simulink model "W09_1_vrx"  (R2024b)
settings: Solver=FixedStepDiscrete  StartTime=0.0  StopTime=inf  FixedStep=Ts_ctrl  RelTol=1e-3
values from neighbouring files (symbols this model uses):
  animate = 0    [W07_compare.m]    (also in W07_crab_demo.m; W07_lookahead_demo.m; W07_setup.m = 1; W09_setup.m = 1)
  crab_comp = 1    [W09_setup.m]
  Delta = DELTAS(i)    [W07_lookahead_demo.m]    (also in W07_setup.m = 10; W09_setup.m = 10)
  F_max = 500    [W07_setup.m]    (also in W09_setup.m)
  half_beam = 1.027135    [W07_setup.m]    (also in W09_setup.m)
  k_prop = 1000 * 0.004422 * 0.2^4    (= 0.0070752)    [W07_setup.m]    (also in W09_setup.m)
  Kd_psi = 200    [W07_setup.m]    (also in W09_setup.m)
  Ki_u = 100    [W07_setup.m]    (also in W09_setup.m)
  Kp_psi = 400    [W07_setup.m]    (also in W09_setup.m)
  Kp_u = 300    [W07_setup.m]    (also in W09_setup.m)
  loiter_radius = 18    [W09_setup.m]
  loiter_turns = 2    [W09_setup.m]
  loiter_wp = 3    [W09_setup.m]
  loiter_xc = wp_north(loiter_wp)    [W09_setup.m]
  loiter_yc = wp_east(loiter_wp)    [W09_setup.m]
  n_max = sqrt(F_max / k_prop)    [W07_setup.m]    (also in W09_setup.m)
  origin_east = -532    [W07_setup.m]    (also in W09_setup.m)
  origin_north = 162    [W07_setup.m]    (also in W09_setup.m)
  p_c = 0.313    [W09_setup.m]
  R_LOS = 5    [W07_lookahead_demo.m]    (also in W07_setup.m; W09_setup.m)
  tau_n = 0.30    (= 0.3)    [W07_setup.m]    (also in W09_setup.m)
  Ts_ctrl = 0.05    [W07_setup.m]    (also in W09_setup.m)
  u_ref = 1.5    [W07_setup.m]    (also in W09_setup.m)
  wp_east = [  20   20  100  100   20 ]    [W07_setup.m]    (also in W09_setup.m = [  20   20   55   90   90 ])
  wp_north = [ -20   60   60  -20  -20 ]    [W07_setup.m]    (also in W09_setup.m = [ -20   50   20   50  -20 ])
libraries: ros2lib x5, slpidlib x1
settings Model: Creator=admin  LastModifiedBy=admin

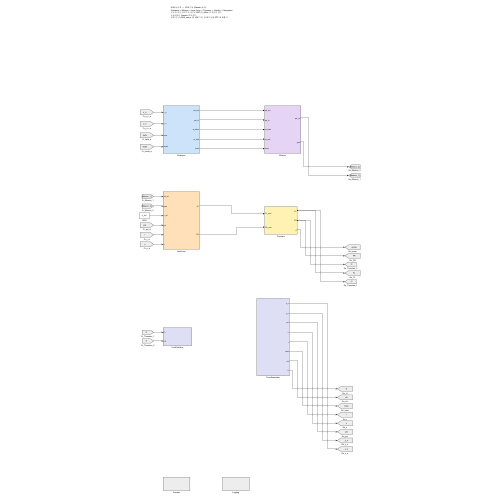
[thumbnail: Simulink's stored preview of the top-level diagram]
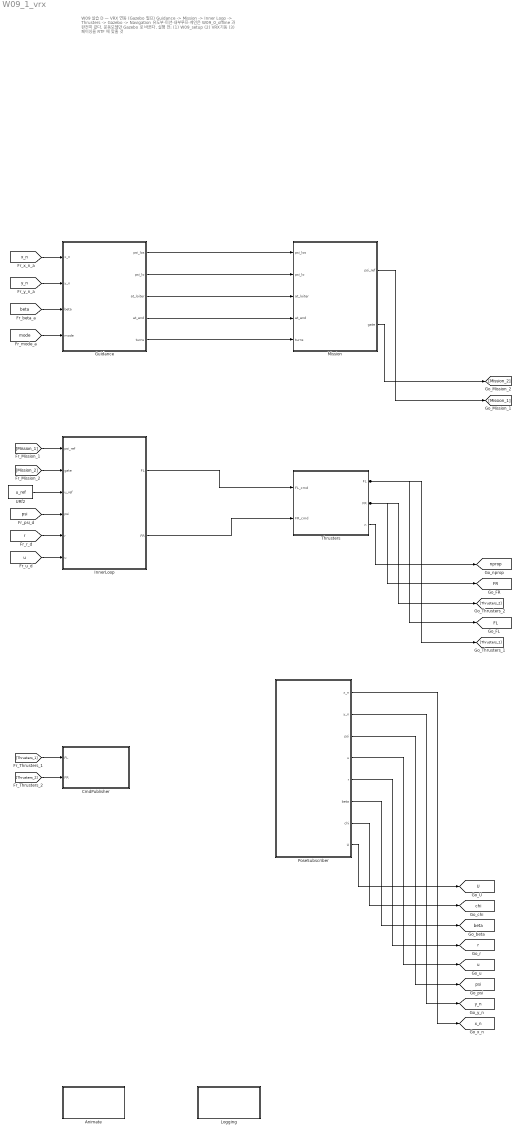
== system W09_1_vrx ==
  note: W09 실습 D  —  VRX 연동 (Gazebo 필요)
      | Guidance -> Mission -> Inner Loop -> Thrusters -> Gazebo -> Navigation
      | 유도부·미션·내부루프·게인은 W09_0_offline 과 완전히 같다.
      | 운동모델만 Gazebo 로 바뀐다.
      | 실행 전: (1) W09_setup  (2) VRX 기동  (3) 페이싱을 RTF 에 맞출 것
  Animate : Subsystem
  CmdPublisher : Subsystem
  Guidance : Subsystem
  InnerLoop : Subsystem
  Logging : Subsystem
  Mission : Subsystem
  PoseSubscriber : Subsystem
  Thrusters : Subsystem
  URf2 : Constant  Value=u_ref
  tag scope: FL=global, FR=global, U=global, beta=global, chi=global, nprop=global, psi=global, r=global, u=global, x_n=global, y_n=global
  wires:
  PoseSubscriber/8(U) -> [U]
  PoseSubscriber/7(chi) -> [chi]
  PoseSubscriber/6(beta) -> [beta]
  PoseSubscriber/5(r) -> [r]
  PoseSubscriber/4(u) -> [u]
  PoseSubscriber/3(psi) -> [psi]
  PoseSubscriber/2(y_n) -> [y_n]
  PoseSubscriber/1(x_n) -> [x_n]
  Thrusters/3(n) -> [nprop]
  Thrusters/2(FR) -> [FR], [Thrusters_2]
  Thrusters/1(FL) -> [FL], [Thrusters_1]
  InnerLoop/2(FR) -> Thrusters/2(FR_cmd)
  InnerLoop/1(FL) -> Thrusters/1(FL_cmd)
  [u] -> InnerLoop/6(u)
  [r] -> InnerLoop/5(r)
  [psi] -> InnerLoop/4(psi)
  URf2/1 -> InnerLoop/3(u_ref)
  Mission/2(gate) -> [Mission_2]
  Mission/1(psi_ref) -> [Mission_1]
  Guidance/5(turns) -> Mission/5(turns)
  Guidance/4(at_end) -> Mission/4(at_end)
  Guidance/3(at_loiter) -> Mission/3(at_loiter)
  Guidance/2(psi_lo) -> Mission/2(psi_lo)
  Guidance/1(psi_los) -> Mission/1(psi_los)
  [mode] -> Guidance/4(mode)
  [beta] -> Guidance/3(beta)
  [y_n] -> Guidance/2(y_n)
  [x_n] -> Guidance/1(x_n)
  [Thrusters_2] -> CmdPublisher/2(FR)
  [Thrusters_1] -> CmdPublisher/1(FL)
  [Mission_2] -> InnerLoop/2(gate)
  [Mission_1] -> InnerLoop/1(psi_ref)

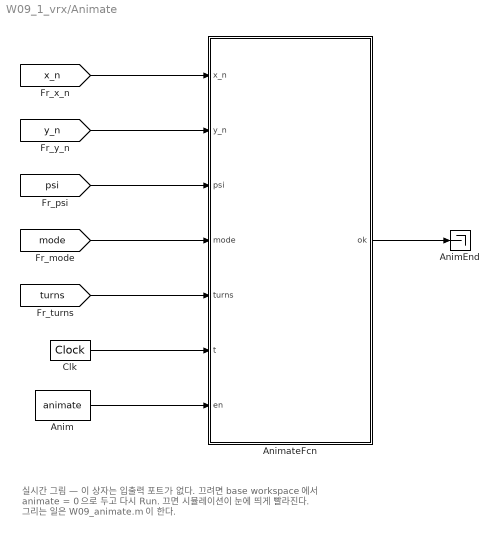
== system W09_1_vrx/Animate ==
  note: 실시간 그림 — 이 상자는 입출력 포트가 없다.
      | 끄려면 base workspace 에서  animate = 0  으로 두고 다시 Run.
      | 끄면 시뮬레이션이 눈에 띄게 빨라진다.
      | 그리는 일은 W09_animate.m 이 한다.
  Anim : Constant  Value=animate
  AnimEnd : Terminator
  AnimateFcn : MATLAB Function  TreatAsAtomicUnit=on
  Clk : DigitalClock  SampleTime=Ts_ctrl
  wires:
  [x_n] -> AnimateFcn/1(x_n)
  [y_n] -> AnimateFcn/2(y_n)
  [psi] -> AnimateFcn/3(psi)
  [mode] -> AnimateFcn/4(mode)
  [turns] -> AnimateFcn/5(turns)
  Clk/1 -> AnimateFcn/6(t)
  Anim/1 -> AnimateFcn/7(en)
  AnimateFcn/1(ok) -> AnimEnd/1

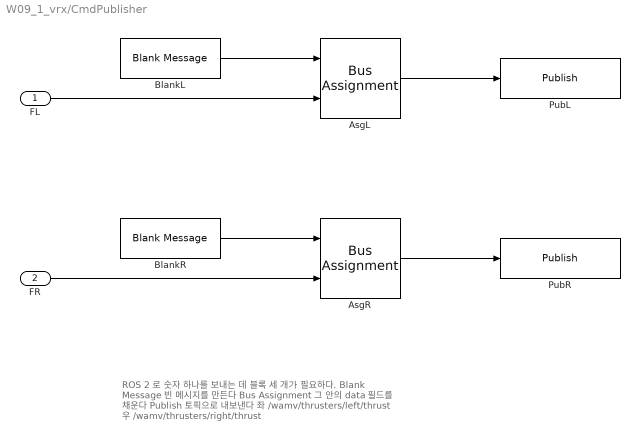
== system W09_1_vrx/CmdPublisher ==
  note: ROS 2 로 숫자 하나를 보내는 데 블록 세 개가 필요하다.
      |   Blank Message   빈 메시지를 만든다
      |   Bus Assignment  그 안의 data 필드를 채운다
      |   Publish         토픽으로 내보낸다
      |
      | 좌 /wamv/thrusters/left/thrust
      | 우 /wamv/thrusters/right/thrust
  FL : Inport
  FR : Inport  Port=2
  AsgL : BusAssignment  AssignedSignals=data
  AsgR : BusAssignment  AssignedSignals=data
  BlankL : ros2lib/Blank Message  messageClass=Message  entityType=std_msgs/Float64  messageType=std_msgs/Float64  SampleTime=Ts_ctrl
  BlankR : ros2lib/Blank Message  messageClass=Message  entityType=std_msgs/Float64  messageType=std_msgs/Float64  SampleTime=Ts_ctrl
  PubL : ros2lib/Publish  topicSource=Specify your own  topic=/wamv/thrusters/left/thrust  messageType=std_msgs/Float64  QOSHistory=Keep last  QOSDepth=1  QOSReliability=Reliable  QOSDurability=Volatile  QOSDeadline=Inf  QOSLifespan=Inf  QOSLiveliness=Automatic  QOSLeaseDuration=Inf  QOSAvoidROSNamespaceConventions=off
  PubR : ros2lib/Publish  topicSource=Specify your own  topic=/wamv/thrusters/right/thrust  messageType=std_msgs/Float64  QOSHistory=Keep last  QOSDepth=1  QOSReliability=Reliable  QOSDurability=Volatile  QOSDeadline=Inf  QOSLifespan=Inf  QOSLiveliness=Automatic  QOSLeaseDuration=Inf  QOSAvoidROSNamespaceConventions=off
  wires:
  BlankL/1 -> AsgL/1
  AsgL/1 -> PubL/1
  FL/1 -> AsgL/2
  BlankR/1 -> AsgR/1
  AsgR/1 -> PubR/1
  FR/1 -> AsgR/2

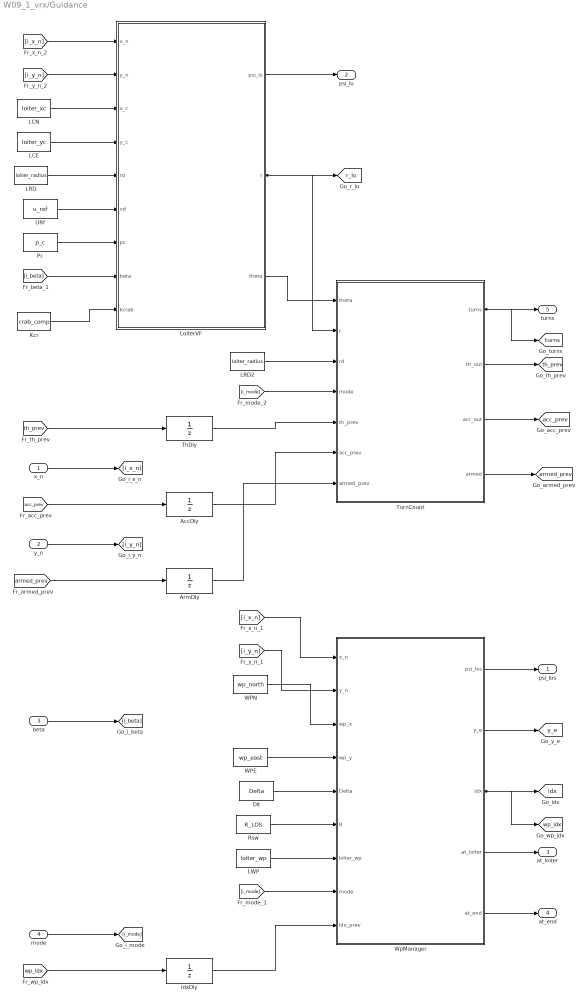
== system W09_1_vrx/Guidance ==
  x_n : Inport
  y_n : Inport  Port=2
  beta : Inport  Port=3
  mode : Inport  Port=4
  AccDly : UnitDelay  SampleTime=Ts_ctrl  HasFrameUpgradeWarning=on
  ArmDly : UnitDelay  SampleTime=Ts_ctrl  HasFrameUpgradeWarning=on
  Dlt : Constant  Value=Delta
  IdxDly : UnitDelay  InitialCondition=1  SampleTime=Ts_ctrl  HasFrameUpgradeWarning=on
  Kcr : Constant  Value=crab_comp
  LCE : Constant  Value=loiter_yc
  LCN : Constant  Value=loiter_xc
  LRD : Constant  Value=loiter_radius
  LRD2 : Constant  Value=loiter_radius
  LWP : Constant  Value=loiter_wp
  LoiterVF : MATLAB Function  TreatAsAtomicUnit=on
  Pc : Constant  Value=p_c
  Rsw : Constant  Value=R_LOS
  ThDly : UnitDelay  SampleTime=Ts_ctrl  HasFrameUpgradeWarning=on
  TurnCount : MATLAB Function  TreatAsAtomicUnit=on
  URf : Constant  Value=u_ref
  WPE : Constant  Value=wp_east
  WPN : Constant  Value=wp_north
  WpManager : MATLAB Function  TreatAsAtomicUnit=on
  psi_los : Outport
  psi_lo : Outport  Port=2
  at_loiter : Outport  Port=3
  at_end : Outport  Port=4
  turns : Outport  Port=5
  tag scope: acc_prev=global, armed_prev=global, idx=global, r_lo=global, th_prev=global, turns=global, wp_idx=global, y_e=global
  wires:
  [i_x_n] -> LoiterVF/1(x_n)
  Pc/1 -> LoiterVF/7(pc)
  y_n/1 -> [i_y_n]
  [i_y_n] -> LoiterVF/2(y_n)
  LCN/1 -> LoiterVF/3(x_c)
  LCE/1 -> LoiterVF/4(y_c)
  LRD/1 -> LoiterVF/5(rd)
  [i_beta] -> LoiterVF/8(beta)
  LRD2/1 -> TurnCount/3(rd)
  URf/1 -> LoiterVF/6(vd)
  AccDly/1 -> TurnCount/6(acc_prev)
  Kcr/1 -> LoiterVF/9(kcrab)
  [th_prev] -> ThDly/1
  x_n/1 -> [i_x_n]
  [acc_prev] -> AccDly/1
  WpManager/3(idx) -> [wp_idx], [idx]
  IdxDly/1 -> WpManager/9(idx_prev)
  [wp_idx] -> IdxDly/1
  [armed_prev] -> ArmDly/1
  beta/1 -> [i_beta]
  mode/1 -> [i_mode]
  WPE/1 -> WpManager/4(wp_y)
  LoiterVF/1(psi_lo) -> psi_lo/1
  LoiterVF/2(r) -> [r_lo], TurnCount/2(r)
  [i_mode] -> WpManager/8(mode)
  LoiterVF/3(theta) -> TurnCount/1(theta)
  [i_mode] -> TurnCount/4(mode)
  ThDly/1 -> TurnCount/5(th_prev)
  ArmDly/1 -> TurnCount/7(armed_prev)
  TurnCount/4(armed) -> [armed_prev]
  [i_x_n] -> WpManager/1(x_n)
  [i_y_n] -> WpManager/2(y_n)
  WPN/1 -> WpManager/3(wp_x)
  Dlt/1 -> WpManager/5(Delta)
  Rsw/1 -> WpManager/6(R)
  TurnCount/1(turns) -> turns/1, [turns]
  LWP/1 -> WpManager/7(loiter_wp)
  TurnCount/2(th_out) -> [th_prev]
  TurnCount/3(acc_out) -> [acc_prev]
  WpManager/1(psi_los) -> psi_los/1
  WpManager/2(y_e) -> [y_e]
  WpManager/4(at_loiter) -> at_loiter/1
  WpManager/5(at_end) -> at_end/1

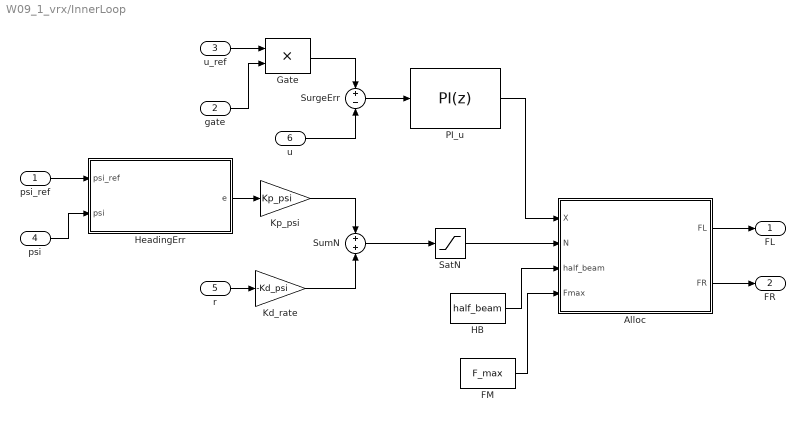
== system W09_1_vrx/InnerLoop ==
  psi_ref : Inport
  gate : Inport  Port=2
  u_ref : Inport  Port=3
  psi : Inport  Port=4
  r : Inport  Port=5
  u : Inport  Port=6
  Alloc : MATLAB Function  TreatAsAtomicUnit=on
  FM : Constant  Value=F_max
  Gate : Product
  HB : Constant  Value=half_beam
  HeadingErr : MATLAB Function  TreatAsAtomicUnit=on
  Kd_rate : Gain  Gain=-Kd_psi
  Kp_psi : Gain  Gain=Kp_psi
  PI_u : slpidlib/PID Controller  Controller=PI  Form=Parallel  TimeDomain=Discrete-time  UseExternalTs=off  SampleTime=Ts_ctrl  IntegratorMethod=Forward Euler  FilterMethod=Forward Euler  ControllerParametersSource=internal  P=Kp_u  I=Ki_u  UseKiTs=off  D=0  UseExternalDerivativeSource=off  N=100  UseFilter=on  TunerSelectOption=Transfer Function Based (PID Tuner App)  InitialConditionSource=internal  InitialConditionForIntegrator=0  InitialConditionForFilter=0  DifferentiatorICPrevScaledInput=0  ExternalReset=none  TrackingMode=off  Kt=1  LimitOutput=on  SatLimitsSource=internal  UpperSaturationLimit=2*F_max  LowerSaturationLimit=-2*F_max  LinearizeAsGain=on  AntiWindupMode=clamping  Kb=1  LimitIntegrator=off  UpperIntegratorSaturationLimit=inf  LowerIntegratorSaturationLimit=-inf  POutMin=[]  POutMax=[]  IOutMin=[]  IOutMax=[]  DOutMin=[]  DOutMax=[]  NOutMin=[]  NOutMax=[]  SumOutMin=[]  SumOutMax=[]  SaturationOutMin=[]  SaturationOutMax=[]  PParamMin=[]  PParamMax=[]  IParamMin=[]  IParamMax=[]  DParamMin=[]  DParamMax=[]  NParamMin=[]  NParamMax=[]  KbParamMin=[]  KbParamMax=[]  KtParamMin=[]  KtParamMax=[]  KbOutMin=[]  KbOutMax=[]  KtOutMin=[]  KtOutMax=[]  IntegratorOutMin=[]  IntegratorOutMax=[]  FilterOutMin=[]  FilterOutMax=[]  SumI1OutMin=[]  SumI1OutMax=[]  SumI2OutMin=[]  SumI2OutMax=[]  SumI3OutMin=[]  SumI3OutMax=[]  SumI4OutMin=[]  SumI4OutMax=[]  SumDOutMin=[]  SumDOutMax=[]  DifferentiatorOutMin=[]  DifferentiatorOutMax=[]  FilterDiffOutCoefMin=[]  FilterDiffOutCoefMax=[]  ReciprocalOutMin=[]  ReciprocalOutMax=[]  SumDenOutMin=[]  SumDenOutMax=[]  SumNumOutMin=[]  SumNumOutMax=[]  DivideOutMin=[]  DivideOutMax=[]  UdiffTsProdOutMin=[]  UdiffTsProdOutMax=[]  NTsProdOutMin=[]  NTsProdOutMax=[]  UintegralTsProdOutMin=[]  UintegralTsProdOutMax=[]  UngainTsProdOutMin=[]  UngainTsProdOutMax=[]  ClampingZeroOutDataTypeStr=Inherit: Inherit via back propagation  ClampingZeroOutMin=[]  ClampingZeroOutMax=[]  FilterDenConstantOutDataTypeStr=Inherit: Inherit via back propagation  FilterDenConstantOutMin=[]  FilterDenConstantOutMax=[]  PCopyOutDataTypeStr=Inherit: Inherit via back propagation  PCopyOutMin=[]  PCopyOutMax=[]  NCopyOutDataTypeStr=Inherit: Inherit via back propagation  NCopyOutMin=[]  NCopyOutMax=[]  IntegratorContinuousStateAttributes=''  IntegratorStateMustResolveToSignalObject=off  IntegratorRTWStateStorageClass=Auto  FilterContinuousStateAttributes=''  FilterStateMustResolveToSignalObject=off  FilterRTWStateStorageClass=Auto  ParallelPVariant=InternalParameters  IdealPVariant=Disabled  IVariant=InternalParameters  DVariant=Disabled  IntegratorVariant=Discrete  SatVariant=Enabled  AWVariant=DiscClampingParallel  PCopyVariant=Disabled  TRVariant=Disabled  FdbkBlocksVariant=Forward  IdealPFdbkVariant=Disabled  SatFdbkVariant=Disabled  DerivativeFilterVariant=Disabled  NVariant=Disabled  NCopyVariant=Disabled_SignalSpec  FilterICVariant=Disabled  IntegratorICVariant=InternalICs  ExternalResetVariant=Disabled  TRSumVariant=Passthrough  SumFdbkVariant=Disabled  SumVariant=Sum_PI  TsampFilterVariant=InternalTs  TsampNgainVariant=Passthrough  TsampIntegralVariant=Disabled_SignalSpec  ExternalSaturationOutDataTypeStr=Inherit: Same as second input  DerivativeSourceVariant=Disabled  PreIntVariant=InternalPreInt
  SatN : Saturate  UpperLimit=2*F_max*half_beam  LowerLimit=-2*F_max*half_beam
  SumN : Sum
  SurgeErr : Sum  Inputs=+-
  FL : Outport
  FR : Outport  Port=2
  wires:
  psi_ref/1 -> HeadingErr/1(psi_ref)
  HeadingErr/1(e) -> Kp_psi/1
  SumN/1 -> SatN/1
  psi/1 -> HeadingErr/2(psi)
  u_ref/1 -> Gate/1
  gate/1 -> Gate/2
  r/1 -> Kd_rate/1
  Gate/1 -> SurgeErr/1
  u/1 -> SurgeErr/2
  Kp_psi/1 -> SumN/1
  Kd_rate/1 -> SumN/2
  SurgeErr/1 -> PI_u/1
  PI_u/1 -> Alloc/1(X)
  SatN/1 -> Alloc/2(N)
  HB/1 -> Alloc/3(half_beam)
  Alloc/2(FR) -> FR/1
  FM/1 -> Alloc/4(Fmax)
  Alloc/1(FL) -> FL/1

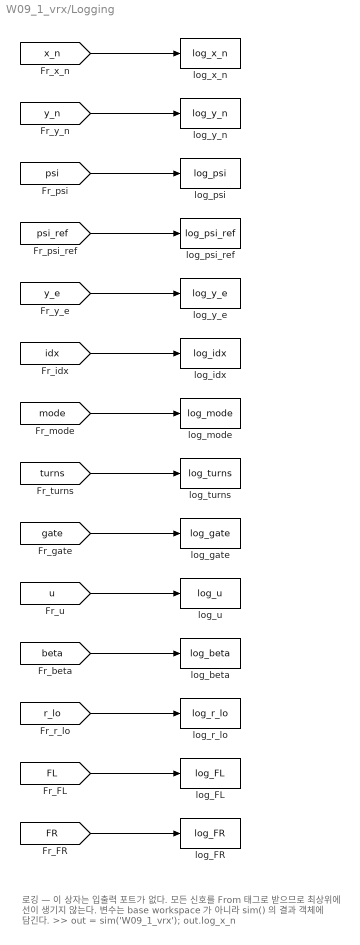
== system W09_1_vrx/Logging ==
  note: 로깅 — 이 상자는 입출력 포트가 없다.
      | 모든 신호를 From 태그로 받으므로 최상위에 선이 생기지 않는다.
      | 변수는 base workspace 가 아니라 sim() 의 결과 객체에 담긴다.
      |   >> out = sim('W09_1_vrx');  out.log_x_n
  log_FL : ToWorkspace  VariableName=log_FL  SaveFormat=Timeseries  SampleTime=Ts_ctrl
  log_FR : ToWorkspace  VariableName=log_FR  SaveFormat=Timeseries  SampleTime=Ts_ctrl
  log_beta : ToWorkspace  VariableName=log_beta  SaveFormat=Timeseries  SampleTime=Ts_ctrl
  log_gate : ToWorkspace  VariableName=log_gate  SaveFormat=Timeseries  SampleTime=Ts_ctrl
  log_idx : ToWorkspace  VariableName=log_idx  SaveFormat=Timeseries  SampleTime=Ts_ctrl
  log_mode : ToWorkspace  VariableName=log_mode  SaveFormat=Timeseries  SampleTime=Ts_ctrl
  log_psi : ToWorkspace  VariableName=log_psi  SaveFormat=Timeseries  SampleTime=Ts_ctrl
  log_psi_ref : ToWorkspace  VariableName=log_psi_ref  SaveFormat=Timeseries  SampleTime=Ts_ctrl
  log_r_lo : ToWorkspace  VariableName=log_r_lo  SaveFormat=Timeseries  SampleTime=Ts_ctrl
  log_turns : ToWorkspace  VariableName=log_turns  SaveFormat=Timeseries  SampleTime=Ts_ctrl
  log_u : ToWorkspace  VariableName=log_u  SaveFormat=Timeseries  SampleTime=Ts_ctrl
  log_x_n : ToWorkspace  VariableName=log_x_n  SaveFormat=Timeseries  SampleTime=Ts_ctrl
  log_y_e : ToWorkspace  VariableName=log_y_e  SaveFormat=Timeseries  SampleTime=Ts_ctrl
  log_y_n : ToWorkspace  VariableName=log_y_n  SaveFormat=Timeseries  SampleTime=Ts_ctrl
  wires:
  [x_n] -> log_x_n/1
  [y_n] -> log_y_n/1
  [psi] -> log_psi/1
  [psi_ref] -> log_psi_ref/1
  [y_e] -> log_y_e/1
  [idx] -> log_idx/1
  [mode] -> log_mode/1
  [turns] -> log_turns/1
  [gate] -> log_gate/1
  [u] -> log_u/1
  [beta] -> log_beta/1
  [r_lo] -> log_r_lo/1
  [FL] -> log_FL/1
  [FR] -> log_FR/1

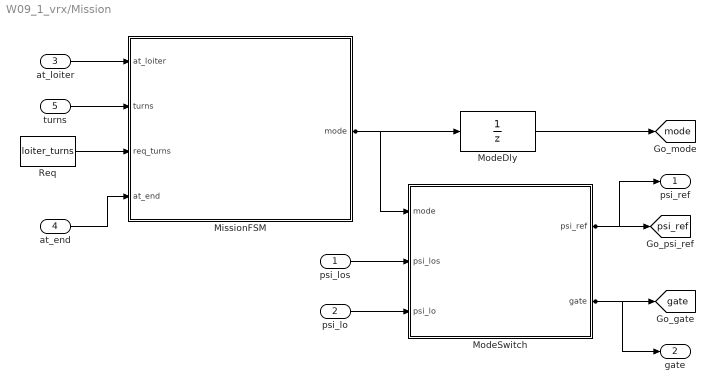
== system W09_1_vrx/Mission ==
  psi_los : Inport
  psi_lo : Inport  Port=2
  at_loiter : Inport  Port=3
  at_end : Inport  Port=4
  turns : Inport  Port=5
  MissionFSM : Stateflow chart  TreatAsAtomicUnit=on
  ModeDly : UnitDelay  InitialCondition=1  SampleTime=Ts_ctrl  HasFrameUpgradeWarning=on
  ModeSwitch : MATLAB Function  TreatAsAtomicUnit=on
  Req : Constant  Value=loiter_turns
  psi_ref : Outport
  gate : Outport  Port=2
  tag scope: gate=global, mode=global, psi_ref=global
  wires:
  at_loiter/1 -> MissionFSM/1(at_loiter)
  turns/1 -> MissionFSM/2(turns)
  Req/1 -> MissionFSM/3(req_turns)
  psi_los/1 -> ModeSwitch/2(psi_los)
  at_end/1 -> MissionFSM/4(at_end)
  psi_lo/1 -> ModeSwitch/3(psi_lo)
  MissionFSM/1(mode) -> ModeSwitch/1(mode), ModeDly/1
  ModeDly/1 -> [mode]
  ModeSwitch/1(psi_ref) -> psi_ref/1, [psi_ref]
  ModeSwitch/2(gate) -> gate/1, [gate]

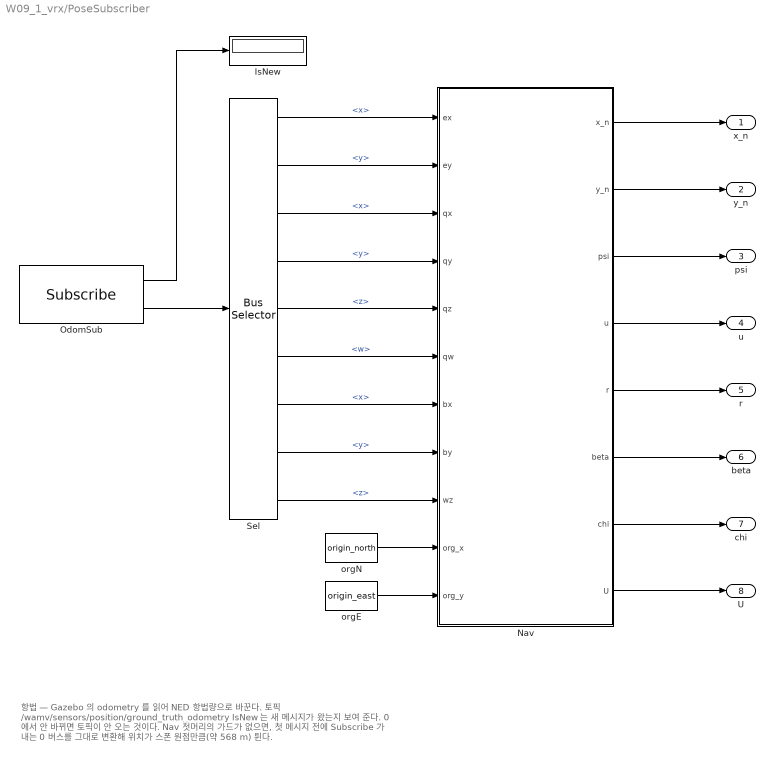
== system W09_1_vrx/PoseSubscriber ==
  note: 항법 — Gazebo 의 odometry 를 읽어 NED 항법량으로 바꾼다.
      |   토픽 /wamv/sensors/position/ground_truth_odometry
      |
      | IsNew 는 새 메시지가 왔는지 보여 준다. 0 에서 안 바뀌면 토픽이 안 오는 것이다.
      | Nav 첫머리의 가드가 없으면, 첫 메시지 전에 Subscribe 가 내는 0 버스를
      | 그대로 변환해 위치가 스폰 원점만큼(약 568 m) 튄다.
  IsNew : Display
  Nav : MATLAB Function  TreatAsAtomicUnit=on
  OdomSub : ros2lib/Subscribe  topicSource=Specify your own  topic=/wamv/sensors/position/ground_truth_odometry  messageType=nav_msgs/Odometry  sampleTime=Ts_ctrl  QOSHistory=Keep last  QOSDepth=1  QOSReliability=Reliable  QOSDurability=Volatile  QOSDeadline=Inf  QOSLifespan=Inf  QOSLiveliness=Automatic  QOSLeaseDuration=Inf  QOSAvoidROSNamespaceConventions=off
  Sel : BusSelector  OutputSignals=pose.pose.position.x,pose.pose.position.y,pose.pose.orientation.x,pose.pose.orientation.y,pose.pose.orientation.z,pose.pose.orientation.w,twist.twist.linear.x,twist.twist.linear.y,twist.twist.angular.z
  orgE : Constant  Value=origin_east
  orgN : Constant  Value=origin_north
  x_n : Outport
  y_n : Outport  Port=2
  psi : Outport  Port=3
  u : Outport  Port=4
  r : Outport  Port=5
  beta : Outport  Port=6
  chi : Outport  Port=7
  U : Outport  Port=8
  wires:
  OdomSub/1 -> IsNew/1
  OdomSub/2 -> Sel/1
  Sel/1 -> Nav/1(ex)  "<x>"
  Sel/2 -> Nav/2(ey)  "<y>"
  Sel/3 -> Nav/3(qx)  "<x>"
  Sel/4 -> Nav/4(qy)  "<y>"
  Sel/5 -> Nav/5(qz)  "<z>"
  Sel/6 -> Nav/6(qw)  "<w>"
  Sel/7 -> Nav/7(bx)  "<x>"
  Sel/8 -> Nav/8(by)  "<y>"
  Sel/9 -> Nav/9(wz)  "<z>"
  orgN/1 -> Nav/10(org_x)
  orgE/1 -> Nav/11(org_y)
  Nav/1(x_n) -> x_n/1
  Nav/2(y_n) -> y_n/1
  Nav/3(psi) -> psi/1
  Nav/4(u) -> u/1
  Nav/5(r) -> r/1
  Nav/6(beta) -> beta/1
  Nav/7(chi) -> chi/1
  Nav/8(U) -> U/1

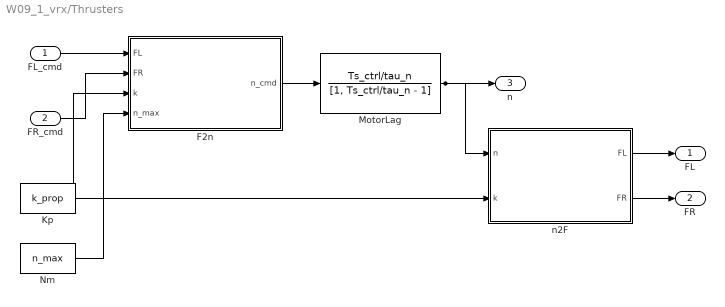
== system W09_1_vrx/Thrusters ==
  FL_cmd : Inport
  FR_cmd : Inport  Port=2
  F2n : MATLAB Function  TreatAsAtomicUnit=on
  Kp : Constant  Value=k_prop
  MotorLag : DiscreteTransferFcn  Numerator=Ts_ctrl/tau_n  Denominator=[1, Ts_ctrl/tau_n - 1]  SampleTime=Ts_ctrl
  Nm : Constant  Value=n_max
  n2F : MATLAB Function  TreatAsAtomicUnit=on
  FL : Outport
  FR : Outport  Port=2
  n : Outport  Port=3
  wires:
  n2F/1(FL) -> FL/1
  Kp/1 -> n2F/2(k), F2n/3(k)
  FR_cmd/1 -> F2n/2(FR)
  FL_cmd/1 -> F2n/1(FL)
  Nm/1 -> F2n/4(n_max)
  F2n/1(n_cmd) -> MotorLag/1
  MotorLag/1 -> n2F/1(n), n/1
  n2F/2(FR) -> FR/1

== matlab function W09_1_vrx/InnerLoop/HeadingErr ==
  data: psi_ref input; e output; psi input
function e = HeadingErr(psi_ref, psi)
%#codegen
% Shortest signed angle, wrapped to [-pi, pi).
d = psi_ref - psi;
e = atan2(sin(d), cos(d));

== matlab function W09_1_vrx/InnerLoop/Alloc ==
  data: X input; FL output; N input; half_beam input; Fmax input; FR output
function [FL, FR] = Alloc(X, N, half_beam, Fmax)
%#codegen
FL = X/2 + N/(2*half_beam);
FR = X/2 - N/(2*half_beam);
if FL >  Fmax, FL =  Fmax; end
if FL < -Fmax, FL = -Fmax; end
if FR >  Fmax, FR =  Fmax; end
if FR < -Fmax, FR = -Fmax; end

== matlab function W09_1_vrx/Thrusters/F2n ==
  data: FL input; n_cmd output; FR input; k input; n_max input
function n_cmd = F2n(FL, FR, k, n_max)
%#codegen
% Inverse propeller law:  F = k*n*|n|  ->  n = sign(F)*sqrt(|F|/k)
F = [FL; FR];
n_cmd = zeros(2,1);
for i = 1:2
    ni = sign(F(i)) * sqrt(abs(F(i))/k);
    if ni >  n_max, ni =  n_max; end
    if ni < -n_max, ni = -n_max; end
    n_cmd(i) = ni;
end

== matlab function W09_1_vrx/Thrusters/n2F ==
  data: n input; FL output; k input; FR output
function [FL, FR] = n2F(n, k)
%#codegen
FL = k * n(1) * abs(n(1));
FR = k * n(2) * abs(n(2));

== matlab function W09_1_vrx/PoseSubscriber/Nav ==
  data: ex input; x_n output; ey input; qx input; qy input; qz input; qw input; bx input; by input; wz input; org_x input; org_y input; y_n output; psi output; u output; r output; beta output; chi output; U output
function [x_n, y_n, psi, u, r, beta, chi, U] = Nav(ex, ey, qx, qy, qz, qw, bx, by, wz, org_x, org_y)
%#codegen
% Gazebo/ROS uses ENU with a body frame of x-forward, y-LEFT, z-UP.
% Marine control uses NED with x-forward, y-STARBOARD, z-DOWN.
% 첫 메시지가 도착하기 전에는 Subscribe 가 0 으로 채운 버스를 낸다.
% 그대로 쓰면 위치가 스폰 원점만큼(약 568 m) 튀어 로그 첫 점이 망가진다.
if ex == 0 && ey == 0
    x_n = 0; y_n = 0; psi = 0; u = 0; r = 0; beta = 0; chi = 0; U = 0;
    return
end
x_n = ey - org_x;
y_n = ex - org_y;
yaw_enu = atan2(2*(qw*qz + qx*qy), 1 - 2*(qy*qy + qz*qz));
p   = pi/2 - yaw_enu;
psi = atan2(sin(p), cos(p));
u = bx;  v = -by;  r = -wz;
U    = sqrt(u*u + v*v);
beta = atan2(v, u);
c    = psi + beta;
chi  = atan2(sin(c), cos(c));

== matlab function W09_1_vrx/Animate/AnimateFcn ==
  data: x_n input; ok output; y_n input; psi input; mode input; turns input; t input; en input
function ok = AnimateFcn(x_n, y_n, psi, mode, turns, t, en)
%#codegen
% Live plot while the model runs. A MATLAB Function block cannot
% plot, so the drawing function is declared extrinsic: Simulink
% calls plain MATLAB instead of generating code for it.
coder.extrinsic('W09_animate');
ok = 1;
if en > 0.5
    W09_animate(x_n, y_n, psi, mode, turns, t);
end

== matlab function W09_1_vrx/Guidance/LoiterVF ==
  data: x_n input; psi_lo output; y_n input; x_c input; y_c input; rd input; vd input; pc input; beta input; kcrab input; r output; theta output
function [psi_lo, r, theta] = LoiterVF(x_n, y_n, x_c, y_c, rd, vd, pc, beta, kcrab)
%#codegen
% Circular-orbit vector field guidance.
%   Jung, Lim, Lee, Bang, "Unmanned Aircraft Vector Field Path Following
%   with Arrival Angle Control", eq. (9) and (13).
%   pc > 0 clockwise, pc < 0 counter-clockwise.

dx = x_n - x_c;
dy = y_n - y_c;
r     = sqrt(dx*dx + dy*dy);
theta = atan2(dy, dx);
if r < 1e-6, r = 1e-6; end

N = sqrt((r - rd)^2 + (pc*r)^2);
if N < 1e-9, N = 1e-9; end
r_dot   = -vd * (r - rd) / N;
rth_dot =  vd * pc * r   / N;

vf_x = r_dot*cos(theta) - rth_dot*sin(theta);
vf_y = r_dot*sin(theta) + rth_dot*cos(theta);

chi_d  = atan2(vf_y, vf_x);
p      = chi_d - kcrab*beta;
psi_lo = atan2(sin(p), cos(p));

== matlab function W09_1_vrx/Guidance/WpManager ==
  data: x_n input; psi_los output; y_n input; wp_x input; wp_y input; Delta input; R input; loiter_wp input; mode input; idx_prev input; y_e output; idx output; at_loiter output; at_end output
function [psi_los, y_e, idx, at_loiter, at_end] = WpManager( ...
         x_n, y_n, wp_x, wp_y, Delta, R, loiter_wp, mode, idx_prev)
%#codegen
% Waypoint bookkeeping plus LOS guidance (week 7).
%   idx = index of the leg START. The leg runs wp(idx) -> wp(idx+1).
%   The index only advances while the mission is in waypoint mode,
%   so a loiter never makes the boat skip a leg.

n = numel(wp_x);
k = min(max(idx_prev, 1), n-1);

xk  = wp_x(k);    yk  = wp_y(k);
xk1 = wp_x(k+1);  yk1 = wp_y(k+1);

pi_p = atan2(yk1 - yk, xk1 - xk);
y_e  = -(x_n - xk)*sin(pi_p) + (y_n - yk)*cos(pi_p);
psi_los = pi_p - atan(y_e / Delta);

d_next  = sqrt((xk1 - x_n)^2 + (yk1 - y_n)^2);
reached = d_next <= R;

% arriving at the loiter waypoint, and arriving at the last one
if reached && ((k+1) == loiter_wp)
    at_loiter = 1;
else
    at_loiter = 0;
end
if reached && (k == n-1)
    at_end = 1;
else
    at_end = 0;
end

% advance only in waypoint mode
if (mode < 1.5) && reached && (k < n-1)
    idx = k + 1;
else
    idx = k;
end

== matlab function W09_1_vrx/Guidance/TurnCount ==
  data: theta input; turns output; r input; rd input; mode input; th_prev input; acc_prev input; armed_prev input; th_out output; acc_out output; armed output
function [turns, th_out, acc_out, armed] = TurnCount( ...
         theta, r, rd, mode, th_prev, acc_prev, armed_prev)
%#codegen
% Count laps, but only while the mission is loitering (mode 2).
% Leaving loiter mode resets the counter, so a second loiter later
% starts from zero again.

th_out = theta;

if mode < 1.5 || mode > 2.5
    turns = 0; acc_out = 0; armed = 0;
    return
end

tol = 0.3*rd;                     % same band as week 8
if armed_prev < 0.5
    acc_out = 0;
    if abs(r - rd) <= tol
        armed = 1;
    else
        armed = 0;
    end
else
    armed = 1;
    d = theta - th_prev;
    d = atan2(sin(d), cos(d));
    acc_out = acc_prev + d;
end
turns = abs(acc_out) / (2*pi);

== stateflow chart W09_1_vrx/Mission/MissionFSM ==
  settings: updateMethod=DISCRETE  sampleTime=Ts_ctrl
  state WpFollow
    en: mode = 1;
  state Finish
    en: mode = 3;
  state Loiter
    en: mode = 2;
  (default) -> WpFollow
  Loiter -> WpFollow : [turns >= req_turns]
  WpFollow -> Finish [order 2] : [at_end > 0.5]
  WpFollow -> Loiter [order 1] : [at_loiter > 0.5]
  data: at_loiter input; turns input; req_turns input; at_end input; mode output

== matlab function W09_1_vrx/Mission/ModeSwitch ==
  data: mode input; psi_ref output; psi_los input; psi_lo input; gate output
function [psi_ref, gate] = ModeSwitch(mode, psi_los, psi_lo)
%#codegen
% Pick the heading command that belongs to the current mission state.
%   mode 1  waypoint following  -> LOS
%   mode 2  loitering           -> vector field
%   mode 3  finished            -> stop
if mode > 2.5
    psi_ref = psi_los;
    gate    = 0;
elseif mode > 1.5
    psi_ref = psi_lo;
    gate    = 1;
else
    psi_ref = psi_los;
    gate    = 1;
end
